simulink model "Position_Sensor_Characteristics"  (R2018a)
settings: Solver=FixedStepDiscrete  StartTime=0.0  StopTime=1  RelTol=1e-3
settings Model: Creator=Choaib ELMADI  LastModifiedBy=Choaib ELMADI
settings OptimizationCC: DefaultParameterBehavior=Inlined  UseDivisionForNetSlopeComputation=on  UseFloatMulNetSlope=on  InlineInvariantSignals=on  PassReuseOutputArgsAs=Individual arguments  ZeroExternalMemoryAtStartup=off  ZeroInternalMemoryAtStartup=off  NoFixptDivByZeroProtection=on  EfficientFloat2IntCast=on  LifeSpan=1  OptimizeBlockOrder=speed  DifferentSizesBufferReuse=on
settings DebuggingCC: ParameterTunabilityLossMsg=error
settings HardwareCC: ProdBitPerPointer=32  ProdBitPerSizeT=32  ProdBitPerPtrDiffT=32  ProdLargestAtomicInteger=Long  ProdLargestAtomicFloat=Double  ProdWordSize=32  ProdLongLongMode=on  ProdHWDeviceType=ARM Compatible->ARM Cortex
settings SFSimCC: MATLABDynamicMemAlloc=off
settings RTWCC: SystemTargetFile=ert.tlc  TemplateMakefile=ert_default_tmf  GenerateReport=on  IncludeHyperlinkInReport=on  LaunchReport=on  GenerateTraceInfo=on  GenerateTraceReport=on  GenerateTraceReportSl=on  GenerateTraceReportSf=on  GenerateTraceReportEml=on  GenerateCodeMetricsReport=on
settings CodeAppCC: ForceParamTrailComments=on  IgnoreCustomStorageClasses=off  OperatorAnnotations=on  SimulinkDataObjDesc=on  SFDataObjDesc=on  CustomSymbolStrGlobalVar=rt$N$M  CustomSymbolStrType=$N$M  CustomSymbolStrFcn=$N$M$F  CustomSymbolStrMacro=$N$M  InsertBlockDesc=on
settings ERTTargetCC: TargetLangStandard=C99 (ISO)  GenerateSampleERTMain=on  IncludeMdlTerminateFcn=off  CombineSignalStateStructs=on  SuppressErrorStatus=on  SupportAbsoluteTime=off  SupportComplex=off  InlinedParameterPlacement=NonHierarchical  ERTCustomFileTemplate=example_file_process.tlc  ERTFilePackagingFormat=CompactWithDataFile

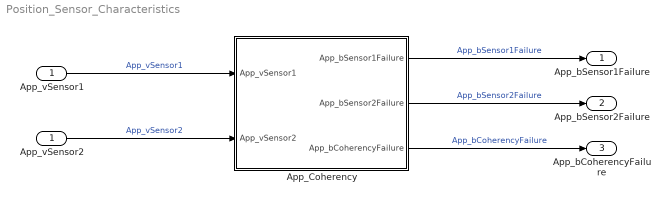
== system Position_Sensor_Characteristics ==
  App_vSensor1 : Inport
  App_Coherency : Subsystem  TreatAsAtomicUnit=on
      settings: RTWSystemCode=Nonreusable function
  App_vSensor2 : InportShadow
  App_bSensor1Failure : Outport
  App_bSensor2Failure : Outport  Port=2
  App_bCoherencyFailure : Outport  Port=3
  wires:
  App_Coherency/1(App_bSensor1Failure) -> App_bSensor1Failure/1  "App_bSensor1Failure"
  App_Coherency/2(App_bSensor2Failure) -> App_bSensor2Failure/1  "App_bSensor2Failure"
  App_Coherency/3(App_bCoherencyFailure) -> App_bCoherencyFailure/1  "App_bCoherencyFailure"
  App_vSensor1/1 -> App_Coherency/1(App_vSensor1)  "App_vSensor1"
  App_vSensor2/1 -> App_Coherency/2(App_vSensor2)  "App_vSensor2"

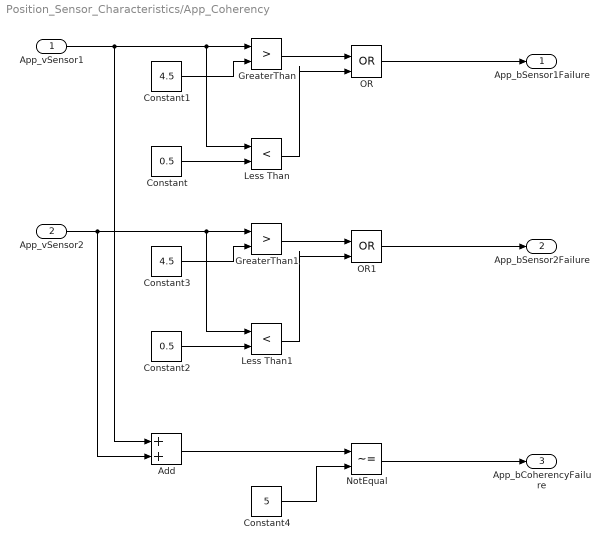
== system Position_Sensor_Characteristics/App_Coherency ==
  App_vSensor1 : Inport
  App_vSensor2 : Inport  Port=2
  Add : Sum
  Constant : Constant  Value=0.5
  Constant1 : Constant  Value=4.5
  Constant2 : Constant  Value=0.5
  Constant3 : Constant  Value=4.5
  Constant4 : Constant  Value=5
  GreaterThan : RelationalOperator  Operator=>  OutDataTypeStr=boolean  RndMeth=Simplest
  GreaterThan1 : RelationalOperator  Operator=>  OutDataTypeStr=boolean  RndMeth=Simplest
  Less Than : RelationalOperator  Operator=<  OutDataTypeStr=boolean  RndMeth=Simplest
  Less Than1 : RelationalOperator  Operator=<  OutDataTypeStr=boolean  RndMeth=Simplest
  NotEqual : RelationalOperator  Operator=~=  OutDataTypeStr=boolean  RndMeth=Simplest
  OR : Logic  Operator=OR  IconShape=distinctive  AllPortsSameDT=off  OutDataTypeStr=boolean
  OR1 : Logic  Operator=OR  IconShape=distinctive  AllPortsSameDT=off  OutDataTypeStr=boolean
  App_bSensor1Failure : Outport
  App_bSensor2Failure : Outport  Port=2
  App_bCoherencyFailure : Outport  Port=3
  wires:
  App_vSensor1/1 -> Add/1, Less Than/1, GreaterThan/1
  OR/1 -> App_bSensor1Failure/1
  GreaterThan/1 -> OR/1
  Less Than/1 -> OR/2
  Constant1/1 -> GreaterThan/2
  Constant/1 -> Less Than/2
  Constant2/1 -> Less Than1/2
  Constant3/1 -> GreaterThan1/2
  Less Than1/1 -> OR1/2
  GreaterThan1/1 -> OR1/1
  OR1/1 -> App_bSensor2Failure/1
  App_vSensor2/1 -> Add/2, GreaterThan1/1, Less Than1/1
  Add/1 -> NotEqual/1
  NotEqual/1 -> App_bCoherencyFailure/1
  Constant4/1 -> NotEqual/2
